simulink model "IW_Motor_0"  (R2020a)
settings: Solver=FixedStepAuto  StartTime=0.0  StopTime=inf  RelTol=1e-3  EnableMultiTasking=on
libraries: mkrmotorcarrierlib x2, eeGeneralControl x1
settings Model: SILPILModeSetting=veronly  ExtModeTrigDuration=2  Creator=bkhusain  LastModifiedBy=mmarathe
settings OptimizationCC: EnhancedBackFolding=on  PassReuseOutputArgsAs=Individual arguments  ZeroExternalMemoryAtStartup=off  ZeroInternalMemoryAtStartup=off  MaxStackSize=64  OptimizeBlockOrder=speed  DifferentSizesBufferReuse=on  OptimizationCustomize=off  EfficientTunableParamExpr=on
settings DebuggingCC: ParameterTunabilityLossMsg=error
settings HardwareCC: ProdBitPerPointer=32  ProdBitPerSizeT=32  ProdBitPerPtrDiffT=32  ProdLargestAtomicInteger=Long  ProdLargestAtomicFloat=Double  ProdWordSize=32  ProdHWDeviceType=ARM Compatible->ARM Cortex
settings SFSimCC: MATLABDynamicMemAlloc=off
settings RTWCC: SystemTargetFile=ert.tlc  HardwareBoard=Arduino Nano 33 IoT  TLCOptions=-aInlineSetEventsForThisBaseRateFcn=TLC_FALSE -aSuppressMultiTaskScheduler=TLC_FALSE -aRateBasedStepFcn=1  TemplateMakefile=ert_default_tmf  Toolchain=Arduino ARM  BuildConfiguration=Faster Runs
settings CodeAppCC: ForceParamTrailComments=on  IgnoreCustomStorageClasses=off  OperatorAnnotations=on  SimulinkDataObjDesc=on  SFDataObjDesc=on  InsertBlockDesc=on
settings ERTTargetCC: SupportContinuousTime=on  SupportVariableSizeSignals=on  ExtModeStaticAllocSize=8192

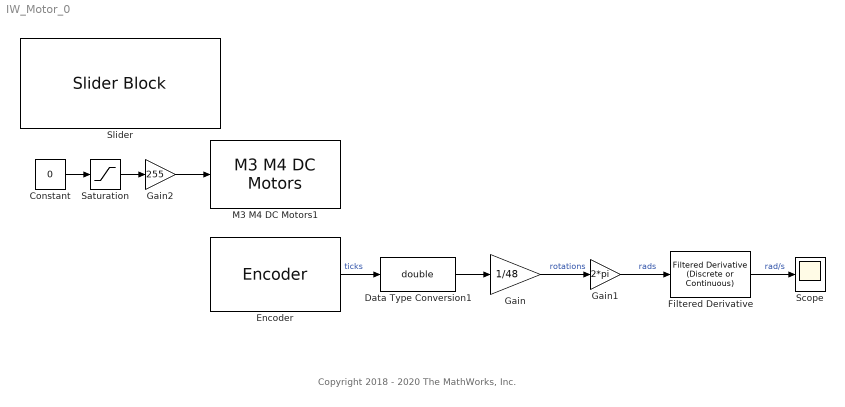
== system IW_Motor_0 ==
  note: Copyright 2018 - 2020 The MathWorks, Inc.
  Constant : Constant  Value=0  SampleTime=0.01
  Data Type Conversion1 : DataTypeConversion  OutDataTypeStr=double
  Encoder : mkrmotorcarrierlib/Encoder  SlaveAddress=uint8( hex2dec( '66' ) )  blockPlatform=ARDUINO  Encoder=1  ShowSpeed=off  ResetOption=on  SampleTime=0.01
      settings: SourceProductName=Simulink Support for Arduino MKR Motor Carrier
  "Filtered Derivative " : eeGeneralControl/Filtered Derivative (Discrete or Continuous)  K=1  T=0.1  B=inf  A=-inf  minRatio=10  init_option=Inherited from block input  x0=0  Ts=0.01
      settings: SourceProductBaseCode=PS
  Gain : Gain  Gain=1/48
  Gain1 : Gain  Gain=2*pi
  Gain2 : Gain  Gain=255
  M3 M4 DC Motors1 : mkrmotorcarrierlib/M3 M4 DC Motors  MotorNumber=M3  forwardPinNumber=2  reversePinNumber=3
      settings: SourceProductBaseCode=ARDUINO
  Saturation : Saturate  UpperLimit=1  LowerLimit=-1
  Scope : Scope
  Slider : SliderBlock  ScaleMin=-1  ScaleMax=1
  wires:
  "Filtered Derivative "/1 -> Scope/1  "rad/s"
  Gain/1 -> Gain1/1  "rotations"
  Gain1/1 -> "Filtered Derivative "/1  "rads"
  Encoder/1 -> Data Type Conversion1/1  "ticks"
  Data Type Conversion1/1 -> Gain/1
  Gain2/1 -> M3 M4 DC Motors1/1
  Constant/1 -> Saturation/1
  Saturation/1 -> Gain2/1
